simulink model "z_one_dive_b"  (R2014a)
settings: Solver=ode45  StartTime=0.0  StopTime=158*3  RelTol=1e-3
values from neighbouring files (symbols this model uses):
  Sample_Time = 1    [main.m]
settings Model: Creator=User  LastModifiedBy=User

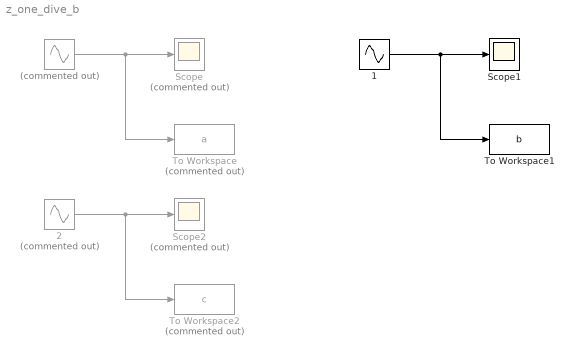
== system z_one_dive_b ==
  " " : Sin  Commented=on  Amplitude=.49  Bias=.5  Frequency=.04  Phase=-1.57  SampleTime=Sample_Time
  " 1" : Sin  Amplitude=.25  Bias=.65  Frequency=.04  Phase=1.57  SampleTime=Sample_Time
  " 2" : Sin  Commented=on  Amplitude=.49  Bias=.5  Frequency=.04  Phase=1.57  SampleTime=Sample_Time
  Scope : Scope  Commented=on
  Scope1 : Scope
  Scope2 : Scope  Commented=on
      settings: SaveName=ScopeData2
  To Workspace : ToWorkspace  Commented=on  VariableName=a  SampleTime=-1
  To Workspace1 : ToWorkspace  VariableName=b  SampleTime=-1
  To Workspace2 : ToWorkspace  Commented=on  VariableName=c  SampleTime=-1
  wires:
  " "/1 -> To Workspace/1, Scope/1
  " 1"/1 -> Scope1/1, To Workspace1/1
  " 2"/1 -> Scope2/1, To Workspace2/1
